simulink model "test13"  (R2021a)
settings: Solver=VariableStepAuto  StartTime=0.0  StopTime=8  RelTol=1e-3
model workspace (MAT data in the model file):
  params = climate_p
  params.A_f = 3100.00212382
  params.A_c = 3299.99831764
  params.minWindows = 0.499999921997
  params.alpha_i = 0.106667779901
  params.cd_c = 8999.32112543
  params.T_ss = 280.000272426
values from neighbouring files (symbols this model uses):
  T_max_heater = 273.15 + 20    (= 293.15)    [test13_script.m]
  T_start_heater = 273.15 + 10    (= 283.15)    [test13_script.m]
libraries: HORTISIM x5
settings Model: SimulationMode=accelerator  OrderedModelArguments=off  Creator=djoroya  LastModifiedBy=djoroya
settings DebuggingCC: UnconnectedInputMsg=none  UnconnectedOutputMsg=none  UnconnectedLineMsg=none

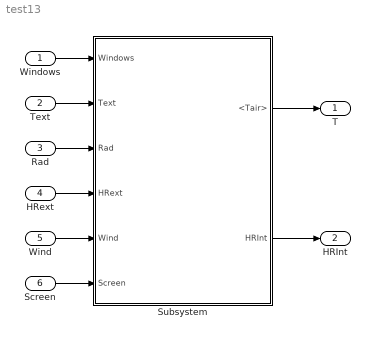
== system test13 ==
  Windows : Inport
  Text : Inport  Port=2
  Rad : Inport  Port=3
  HRext : Inport  Port=4
  Wind : Inport  Port=5
  Screen : Inport  Port=6
  Subsystem : Subsystem
  T : Outport
  HRInt : Outport  Port=2
  wires:
  Subsystem/1(<Tair>) -> T/1
  Windows/1 -> Subsystem/1(Windows)
  Text/1 -> Subsystem/2(Text)
  Rad/1 -> Subsystem/3(Rad)
  HRext/1 -> Subsystem/4(HRext)
  Wind/1 -> Subsystem/5(Wind)
  Subsystem/2(HRInt) -> HRInt/1
  Screen/1 -> Subsystem/6(Screen)

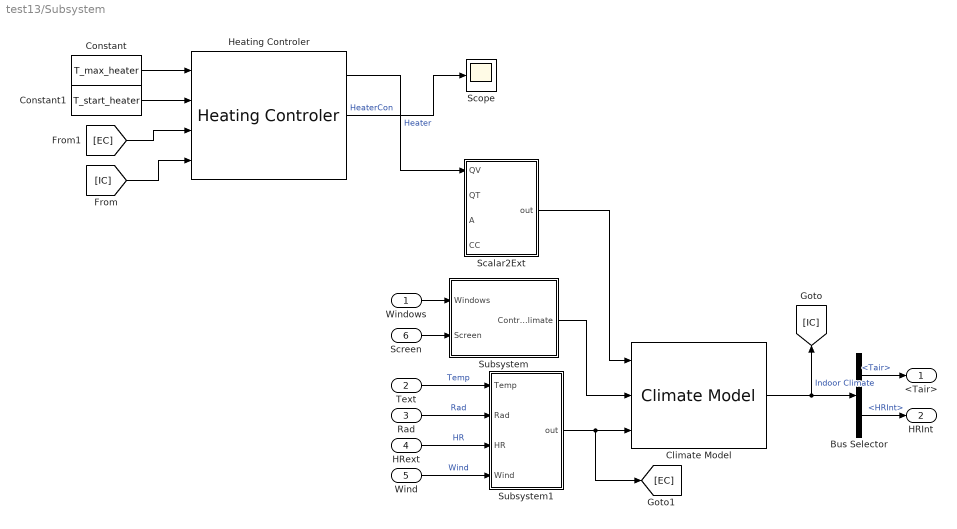
== system test13/Subsystem ==
  Windows : Inport
  Text : Inport  Port=2
  Rad : Inport  Port=3
  HRext : Inport  Port=4
  Wind : Inport  Port=5
  Screen : Inport  Port=6
  Bus Selector : BusSelector  OutputSignals=Temp.Tair,Gas.HRInt
  Climate Model : HORTISIM/Climate/Models/Climate Model  params=climate_params  x0=cic
      settings: SourceProductName=Horti Simulator
  Constant : Constant  Value=T_max_heater
  Constant1 : Constant  Value=T_start_heater
  Heating Controler : HORTISIM/Climate/Controls/Heating Controler  params=heat_p  x0=heat_ic
      settings: SourceProductName=Horti Simulator
  Scalar2Ext : Subsystem
  Scope : Scope
  Subsystem : Subsystem
  Subsystem1 : Subsystem
  <Tair> : Outport
  HRInt : Outport  Port=2
  wires:
  Climate Model/1 -> [IC], Bus Selector/1  "Indoor Climate"
  Bus Selector/1 -> <Tair>/1  "<Tair>"
  Bus Selector/2 -> HRInt/1  "<HRInt>"
  Scalar2Ext/1(out) -> Climate Model/1
  Heating Controler/1 -> Scalar2Ext/1(QV)  "Heater"
  [IC] -> Heating Controler/4
  [EC] -> Heating Controler/3
  Constant/1 -> Heating Controler/1
  Windows/1 -> Subsystem/1(Windows)
  Screen/1 -> Subsystem/2(Screen)
  Subsystem/1(Control Climate) -> Climate Model/2
  Subsystem1/1(out) -> [EC], Climate Model/3
  Text/1 -> Subsystem1/1(Temp)  "Temp"
  Rad/1 -> Subsystem1/2(Rad)  "Rad"
  HRext/1 -> Subsystem1/3(HR)  "HR"
  Wind/1 -> Subsystem1/4(Wind)  "Wind"
  Constant1/1 -> Heating Controler/2
  Heating Controler/2 -> Scope/1  "HeaterCon"

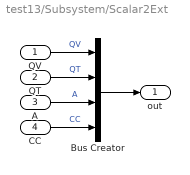
== system test13/Subsystem/Scalar2Ext ==
  QV : Inport
  QT : Inport  Port=2
  A : Inport  Port=3
  CC : Inport  Port=4
  Bus Creator : BusCreator  Inputs=4
  out : Outport
  wires:
  Bus Creator/1 -> out/1
  QV/1 -> Bus Creator/1  "QV"
  QT/1 -> Bus Creator/2  "QT"
  A/1 -> Bus Creator/3  "A"
  CC/1 -> Bus Creator/4  "CC"

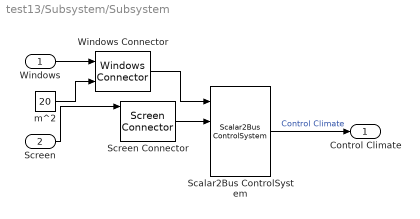
== system test13/Subsystem/Subsystem ==
  Windows : Inport
  Screen : Inport  Port=2
  Scalar2Bus ControlSystem : HORTISIM/Other  Functions/Scalar2Bus  ControlSystem  SystemSampleTime=-1  VariantActivationTime=update diagram  Latency=0  AutoFrameSizeCalculation=off
      settings: SourceProductName=Horti Simulator
  Screen Connector : HORTISIM/Other  Functions/Screen Connector  SystemSampleTime=-1  VariantActivationTime=update diagram  Latency=0  AutoFrameSizeCalculation=off
      settings: SourceProductName=Horti Simulator
  Windows Connector : HORTISIM/Other  Functions/Windows Connector  SystemSampleTime=-1  VariantActivationTime=update diagram  Latency=0  AutoFrameSizeCalculation=off
      settings: SourceProductName=Horti Simulator
  m^2 : Constant  Value=20
  Control Climate : Outport
  wires:
  ? -> Scalar2Bus ControlSystem/3
  ? -> Screen Connector/2
  Scalar2Bus ControlSystem/1 -> Control Climate/1  "Control Climate"
  ? -> Screen Connector/3
  Windows/1 -> Windows Connector/1
  m^2/1 -> Windows Connector/2
  Windows Connector/1 -> Scalar2Bus ControlSystem/1
  ? -> Scalar2Bus ControlSystem/4
  Screen/1 -> Screen Connector/1
  Screen Connector/1 -> Scalar2Bus ControlSystem/2

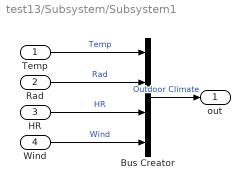
== system test13/Subsystem/Subsystem1 ==
  Temp : Inport
  Rad : Inport  Port=2
  HR : Inport  Port=3
  Wind : Inport  Port=4
  Bus Creator : BusCreator  Inputs=4
  out : Outport
  wires:
  HR/1 -> Bus Creator/3  "HR"
  Wind/1 -> Bus Creator/4  "Wind"
  Temp/1 -> Bus Creator/1  "Temp"
  Rad/1 -> Bus Creator/2  "Rad"
  Bus Creator/1 -> out/1  "Outdoor Climate"
